simulink model "Prob_2_3"  (Simulink 7.7)
settings: Solver=ode45  StartTime=0.0  StopTime=18.5  RelTol=1e-3
settings Model: Creator=srikanth  LastModifiedBy=srikanth

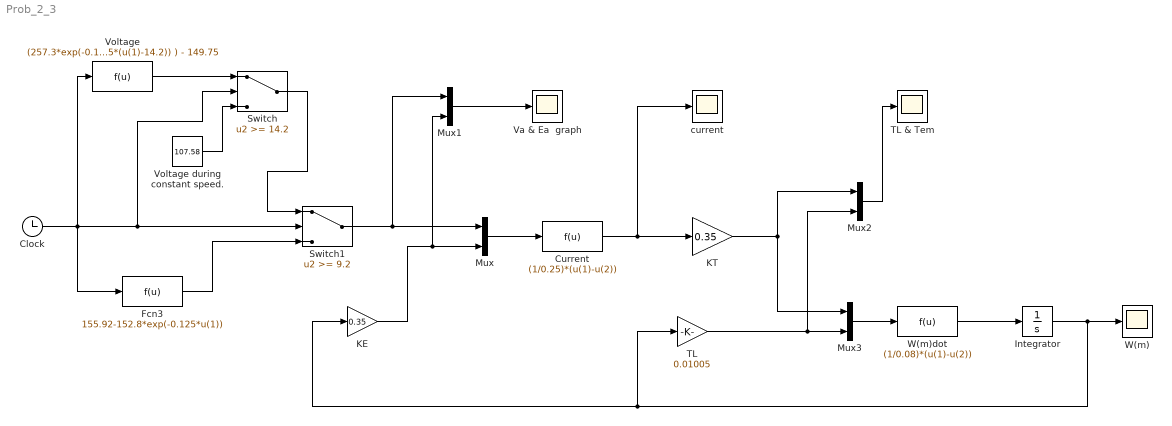
== system Prob_2_3 ==
  Clock : Clock
      settings: Decimation=19
  Current : Fcn  Expr=(1/0.25)*(u(1)-u(2))
  Fcn3 : Fcn  Expr=155.92-152.8*exp(-0.125*u(1))
  Integrator : Integrator
  KE : Gain  Gain=0.35
  KT : Gain  Gain=0.35
  Mux{,1..3} (4 alike) : Mux  Inputs=2
  Switch : Switch  Threshold=14.2
  Switch1 : Switch  Threshold=9.2
  TL : Gain  Gain=0.01005
  TL & Tem : Scope
  Va & Ea  graph : Scope
  Voltage : Fcn  Expr=(257.3*exp(-0.125*(u(1)-14.2)) ) - 149.75
  Voltage during constant speed. : Constant  Value=107.58
  W(m) : Scope
      settings: SaveName=ScopeData3
  W(m)dot : Fcn  Expr=(1/0.08)*(u(1)-u(2))
  current : Scope
      settings: SaveName=ScopeData2
  wires:
  Clock/1 -> Voltage/1, Fcn3/1, Switch1/2, Switch/2
  Fcn3/1 -> Switch1/3
  Voltage/1 -> Switch/1
  Voltage during constant speed./1 -> Switch/3
  Switch/1 -> Switch1/1
  Switch1/1 -> Mux/1, Mux1/1
  KE/1 -> Mux/2, Mux1/2
  Mux/1 -> Current/1
  Current/1 -> KT/1, current/1
  Mux1/1 -> Va & Ea  graph/1
  KT/1 -> Mux2/1, Mux3/1
  TL/1 -> Mux3/2, Mux2/2
  Mux2/1 -> TL & Tem/1
  Mux3/1 -> W(m)dot/1
  W(m)dot/1 -> Integrator/1
  Integrator/1 -> W(m)/1, TL/1, KE/1
